simulink model "SignalModelL6_shim_b"  (R2017a)
settings: Solver=FixedStepAuto  StartTime=0.0  StopTime=20  FixedStep=0.01  RelTol=1e-3
undefined symbols (not defined in the file): k
settings Model: Creator=roman  LastModifiedBy=roman

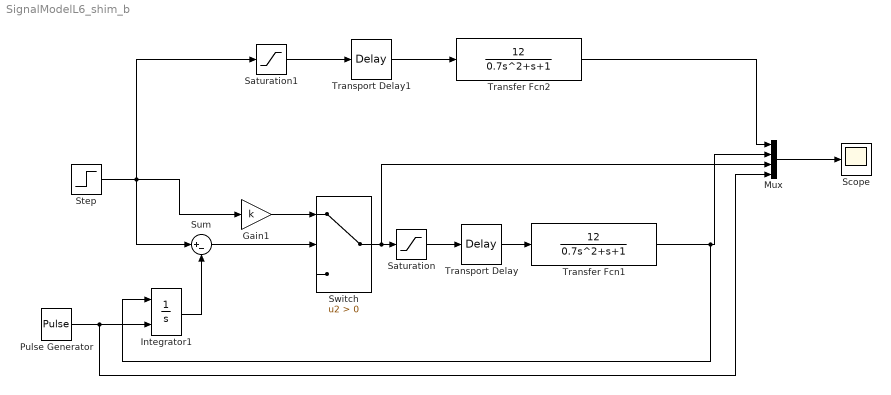
== system SignalModelL6_shim_b ==
  Gain1 : Gain  Gain=k
  Integrator1 : Integrator  ExternalReset=rising
  Mux : Mux
  Pulse Generator : DiscretePulseGenerator  PulseType=Time based  Period=0.1  PulseWidth=50
  Saturation : Saturate  UpperLimit=2000  LowerLimit=-2000
  Saturation1 : Saturate  UpperLimit=2000  LowerLimit=-2000
  Scope : Scope
  Step : Step  Time=0  SampleTime=0
  Sum : Sum  Inputs=|+-
  Switch : Switch  Criteria=u2 > Threshold
  Transfer Fcn1 : TransferFcn  Numerator=[12]  Denominator=[0.7 1 1]
  Transfer Fcn2 : TransferFcn  Numerator=[12]  Denominator=[0.7 1 1]
  Transport Delay : TransportDelay  DelayTime=0.1
  Transport Delay1 : TransportDelay  DelayTime=0.1
  wires:
  Saturation1/1 -> Transport Delay1/1
  Mux/1 -> Scope/1
  Step/1 -> Gain1/1, Sum/1, Saturation1/1
  Transfer Fcn2/1 -> Mux/1
  Saturation/1 -> Transport Delay/1
  Transport Delay/1 -> Transfer Fcn1/1
  Transport Delay1/1 -> Transfer Fcn2/1
  Switch/1 -> Mux/3, Saturation/1
  Gain1/1 -> Switch/1
  Transfer Fcn1/1 -> Integrator1/1, Mux/2
  Pulse Generator/1 -> Mux/4, Integrator1/2
  Integrator1/1 -> Sum/2
  Sum/1 -> Switch/2
